simulink model "robot_sim"  (Simulink 7.5)
settings: Solver=ode45  StartTime=0.0  StopTime=200  RelTol=1e-3
values from neighbouring files (symbols this model uses):
  P = [ps, vs, pe, ve]    [planpath.m]
undefined symbols (not defined in the file or in its folder): drawRobot, flatness, trajectory
settings Model: Creator=rwb5  LastModifiedBy=rwb5
settings DataIOCC: SignalLoggingName=sigsOut
settings OptimizationCC: BooleanDataType=off
settings DebuggingCC: SaveWithParameterizedLinksMsg=none  SignalResolutionControl=TryResolveAllWithWarning  SolverPrmCheckMsg=none  MultiTaskDSMMsg=warning  MultiTaskCondExecSysMsg=none  StrictBusMsg=None
settings HardwareCC: TargetUnknown=on
settings RTWCC: IncludeERTFirstTime=on

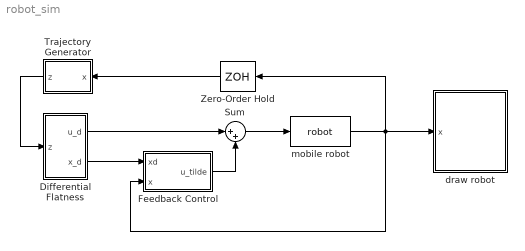
== system robot_sim ==
  Differential Flatness : Subsystem
  Feedback Control : Subsystem
  Sum : Sum  Inputs=|++  OutDataType=fixdt(1, 16)  OutScaling=2^0
  Trajectory Generator : Subsystem
  Zero-Order Hold : ZeroOrderHold  SampleTime=P.Te
  draw robot : Subsystem
      mask Display: image(imread('tv.jpg'))
  mobile robot : S-Function  FunctionName=robot  Parameters=P  EnableBusSupport=off
  wires:
  mobile robot/1 -> draw robot/1(x), Feedback Control/2(x), Zero-Order Hold/1
  Trajectory Generator/1(z) -> Differential Flatness/1(z)
  Sum/1 -> mobile robot/1
  Differential Flatness/1(u_d) -> Sum/1
  Differential Flatness/2(x_d) -> Feedback Control/1(xd)
  Feedback Control/1(u_tilde) -> Sum/2
  Zero-Order Hold/1 -> Trajectory Generator/1(x)

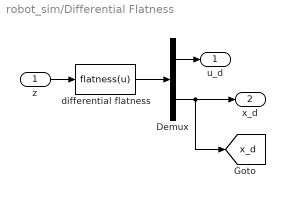
== system robot_sim/Differential Flatness ==
  z : Inport
  Demux : Demux  Outputs=[2;4]
  differential flatness : MATLABFcn  MATLABFcn=flatness(u)  OutputDimensions=6
  u_d : Outport
  x_d : Outport  Port=2
  tag scope: x_d=global
  wires:
  differential flatness/1 -> Demux/1
  Demux/1 -> u_d/1
  z/1 -> differential flatness/1
  Demux/2 -> x_d/1, [x_d]

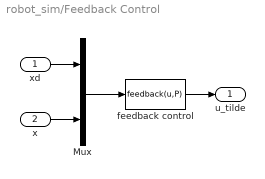
== system robot_sim/Feedback Control ==
  xd : Inport
  x : Inport  Port=2
  Mux : Mux  Inputs=2
  feedback control : MATLABFcn  MATLABFcn=feedback(u,P)  OutputDimensions=2
  u_tilde : Outport
  wires:
  feedback control/1 -> u_tilde/1
  Mux/1 -> feedback control/1
  xd/1 -> Mux/1
  x/1 -> Mux/2

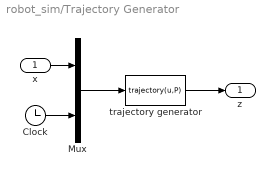
== system robot_sim/Trajectory Generator ==
  x : Inport
  Clock : Clock
      settings: Decimation=10
  Mux : Mux  Inputs=2
  trajectory generator : MATLABFcn  MATLABFcn=trajectory(u,P)  OutputDimensions=6
  z : Outport
  wires:
  trajectory generator/1 -> z/1
  Mux/1 -> trajectory generator/1
  x/1 -> Mux/1
  Clock/1 -> Mux/2

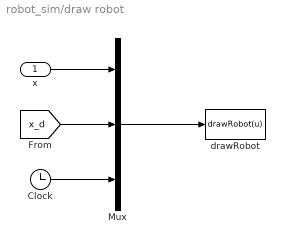
== system robot_sim/draw robot ==
  x : Inport
  Clock : Clock
      settings: Decimation=10
  Mux : Mux  Inputs=3
  drawRobot : MATLABFcn  MATLABFcn=drawRobot(u)  OutputDimensions=0  SampleTime=0.1
  wires:
  Mux/1 -> drawRobot/1
  x/1 -> Mux/1
  Clock/1 -> Mux/3
  [x_d] -> Mux/2
